simulink model "CartPole_env"  (R2023a)
settings: Solver=ode3  StartTime=0.0  StopTime=40  FixedStep=0.02  RelTol=1e-3  EnableMultiTasking=on
InitFcn:
  | Mp = 0.1;
  | Mc = 1;
  | l = 0.5; %half of the pole's length (distance from pivot to the center of mass of the pole)
  | g =9.81;
settings Model: Creator=divij  LastModifiedBy=divij
settings DataIOCC: SaveFormat=Structure
settings OptimizationCC: ZeroExternalMemoryAtStartup=off  ZeroInternalMemoryAtStartup=off
settings DebuggingCC: AlgebraicLoopMsg=none
settings RTWCC: PackageGeneratedCodeAndArtifacts=on  Toolchain=Catkin  BuildConfiguration=Debug  TargetLang=C++
settings GRTTargetCC: TargetLangStandard=C++11 (ISO)  MatFileLogging=off  CodeInterfacePackaging=C++ class

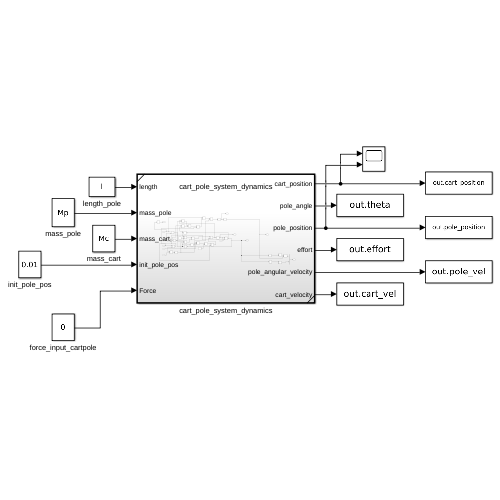
[thumbnail: Simulink's stored preview of the top-level diagram]
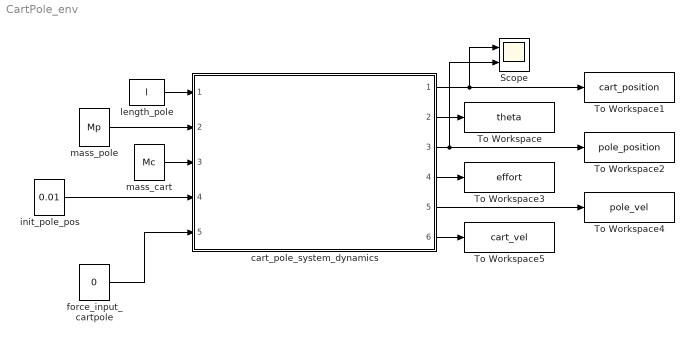
== system CartPole_env ==
  Scope : Scope  NumInputPorts=2
  To Workspace : ToWorkspace  VariableName=theta  SaveFormat=Timeseries  SampleTime=-1
  To Workspace1 : ToWorkspace  VariableName=cart_position  SampleTime=-1
  To Workspace2 : ToWorkspace  VariableName=pole_position  SampleTime=-1
  To Workspace3 : ToWorkspace  VariableName=effort  SaveFormat=Timeseries  SampleTime=-1
  To Workspace4 : ToWorkspace  VariableName=pole_vel  SaveFormat=Timeseries  SampleTime=-1
  To Workspace5 : ToWorkspace  VariableName=cart_vel  SaveFormat=Timeseries  SampleTime=-1
  cart_pole_system_dynamics : Subsystem  TreatAsAtomicUnit=on  ReferencedSubsystem=cart_pole_system_dynamics
      settings: MinAlgLoopOccurrences=on
  force_input_cartpole : Constant  Value=0
  init_pole_pos : Constant  Value=0.01
  length_pole : Constant  Value=l
  mass_cart : Constant  Value=Mc
  mass_pole : Constant  Value=Mp
  wires:
  cart_pole_system_dynamics/1 -> Scope/1, To Workspace1/1
  cart_pole_system_dynamics/2 -> To Workspace/1
  mass_pole/1 -> cart_pole_system_dynamics/2
  length_pole/1 -> cart_pole_system_dynamics/1
  mass_cart/1 -> cart_pole_system_dynamics/3
  cart_pole_system_dynamics/3 -> To Workspace2/1, Scope/2
  cart_pole_system_dynamics/4 -> To Workspace3/1
  force_input_cartpole/1 -> cart_pole_system_dynamics/5
  cart_pole_system_dynamics/5 -> To Workspace4/1
  cart_pole_system_dynamics/6 -> To Workspace5/1
  init_pole_pos/1 -> cart_pole_system_dynamics/4
